simulink model "PolePlacement_Observer_DUE_SISO"  (R2019a)
settings: Solver=FixedStepAuto  StartTime=0.0  StopTime=120  RelTol=1e-3  EnableMultiTasking=on
undefined symbols (not defined in the file): A, B, C, DiscIntNeverNeededParam, i0, K, L, sigbuilder_block, Ts, u0, y0
libraries: arduinolib x1
settings Model: SimulationMode=external  ExtModeTrigDuration=2  Creator=jakub  LastModifiedBy=jakub
settings OptimizationCC: EnhancedBackFolding=on  PassReuseOutputArgsAs=Individual arguments  MaxStackSize=64  OptimizeBlockOrder=speed  DifferentSizesBufferReuse=on  OptimizationCustomize=off
settings DebuggingCC: ParameterTunabilityLossMsg=error
settings HardwareCC: ProdBitPerPointer=32  ProdBitPerSizeT=32  ProdBitPerPtrDiffT=32  ProdLargestAtomicInteger=Long  ProdLargestAtomicFloat=Double  ProdWordSize=32  ProdHWDeviceType=ARM Compatible->ARM Cortex
settings SFSimCC: MATLABDynamicMemAlloc=off
settings RTWCC: SystemTargetFile=ert.tlc  HardwareBoard=Arduino Due  TLCOptions=-aInlineSetEventsForThisBaseRateFcn=TLC_FALSE -aSuppressMultiTaskScheduler=TLC_FALSE -aRateBasedStepFcn=1  TemplateMakefile=ert_default_tmf  GenerateReport=on  Toolchain=Arduino ARM  BuildConfiguration=Faster Runs  IncludeHyperlinkInReport=on  LaunchReport=on  GenerateTraceInfo=on  GenerateTraceReport=on  GenerateTraceReportSl=on  GenerateTraceReportSf=on  GenerateTraceReportEml=on
settings CodeAppCC: ForceParamTrailComments=on  IgnoreCustomStorageClasses=off  OperatorAnnotations=on  SimulinkDataObjDesc=on  SFDataObjDesc=on  InsertBlockDesc=on
settings ERTTargetCC: SupportContinuousTime=on  SupportVariableSizeSignals=on  ExtModeStaticAllocSize=24576

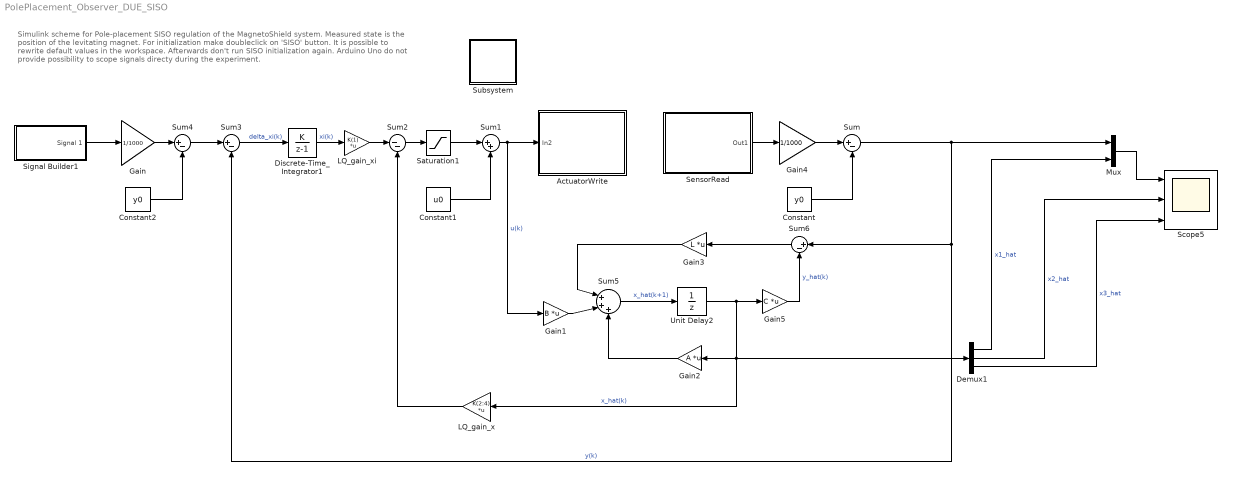
== system PolePlacement_Observer_DUE_SISO ==
  note: Simulink scheme for Pole-placement SISO regulation of the MagnetoShield system. Measured state is the position
      | of the levitating magnet.
      | For initialization make doubleclick on 'SISO' button.
      |
      | It is possible to rewrite default values in the workspace. Afterwards don't run SISO initialization again.
      |
      | Arduino Uno do not provide possibility to scope signals directy during the experiment.
  ActuatorWrite : Subsystem  AncestorBlock=MagnetoLibrary/ActuatorWrite  mask{Board=DUE, Units=Volts}
      mask prompts: Board "Type of the Arduino board"; Units "Input unite"
      mask help:
      | ActuatorWrite block allows to set desired voltage value on the electromagnet.
      | Input signal:
      |  - Voltage - value in range 0 - 12 V
      |  - Percent
      |  - DAC levels - value in range 0 - 4095
      | This block converts input control signal into suficient form (12-bit number) and writes the information on the MCP4725-DAC converter.
      mask init:
      | mask_popup = get_param(gcb,'Board'); % which popup is choosen
      | % path to the I2C Write block
      | system = gcb;
      | way = strcat(system,'/I2C Write UNO');
      | % set Module based on Arduino type
      | if strcmp(mask_popup(1),'U')
      |     set_param(way,'I2CModule','0'); % Uno/Mega - module 0
      | elseif strcmp(mask_popup(1),'D')
      |     set_param(way,'I2CModule','1'); % Due - module 1
      | end
      settings: CopyFcn=set_param(gcb, 'LinkStatus', 'inactive')
      mask TypeOptions Board: UNO/MEGA | DUE
      mask TypeOptions Units: Volts | Percent | DAC levels
      mask DialogControl DescGroupVar Prompt: ActuatorWrite block
      mask DialogControl Container3 Prompt: Arduino board
      mask Display: image('assets\MagnetoFig\ActuatorWrite.svg');
  Constant : Constant  Value=y0
  Constant1 : Constant  Value=u0
  Constant2 : Constant  Value=y0
  Demux1 : Demux  Outputs=3
  Discrete-Time_ Integrator1 : DiscreteIntegrator  IntegratorMethod=Accumulation: Forward Euler  SampleTime=Ts  LimitOutput=on  UpperSaturationLimit=1  LowerSaturationLimit=-1  ICPrevOutput=DiscIntNeverNeededParam  ICPrevScaledInput=DiscIntNeverNeededParam
  Gain : Gain  Gain=1/1000
  Gain1 : Gain  Gain=B  Multiplication=Matrix(K*u)
  Gain2 : Gain  Gain=A  Multiplication=Matrix(K*u)
  Gain3 : Gain  Gain=L  Multiplication=Matrix(K*u)
  Gain4 : Gain  Gain=1/1000
  Gain5 : Gain  Gain=C  Multiplication=Matrix(K*u)
  LQ_gain_x : Gain  Gain=K(2:4)  Multiplication=Matrix(K*u)
  LQ_gain_xi : Gain  Gain=K(1)  Multiplication=Matrix(K*u)
  Mux : Mux  Inputs=2
  Saturation1 : Saturate  UpperLimit=12-u0  LowerLimit=0-u0
  Scope5 : Scope  NumInputPorts=3
  SensorRead : Subsystem  AncestorBlock=MagnetoLibrary/SensorRead  mask{board=DUE, sensor=Distance [mm], sampling=Ts}
      mask prompts: board "Type of the Arduino board"; sensor "Sensor type"; sampling "Sampling period [s]"
      mask help: Output of the block provides data about a choosen quantity measured on the MagnetoShiled device.
      mask init:
      | letter = sensor;
      | if letter==1 % distance
      | path='assets\MagnetoFig\SensorRead\SensorRead_Hall.svg';
      | elseif letter==2 % current
      | path='assets\MagnetoFig\SensorRead\SensorRead_Current.svg';
      | elseif letter==3 % voltage
      | path='assets\MagnetoFig\SensorRead\SensorRead_Voltage.svg';
      | else % reference
      | path='assets\MagnetoFig\SensorRead\Potentiometer.svg';    
      | end
      settings: CopyFcn=set_param(gcb, 'LinkStatus', 'inactive')
      mask TypeOptions board: UNO/MEGA | DUE
      mask TypeOptions sensor: Distance [mm] | Current [mA] | Voltage [V] | Analog reference [%]
      mask Callback sensor:
      | mask_popup = get_param(gcb,'sensor'); % which popup is choosen
      | % path to the I2C Write block
      | system = gcb;
      | way = strcat(system,'/Analog Input');
      | % set Module based on Arduino type
      | if strcmp(mask_popup(1),'D')
      |     set_param(way,'pinNumber','3');
      | elseif strcmp(mask_popup(1),'V')
      |     set_param(way,'pinNumber','1'); % Due - module 1
      | elseif strcmp(mask_popup(1),'C')
      |     set_param(way,'pinNumber','2'); % Due - module 1
      | elseif strcmp(mask_popup(1),'A')
      |     set_param(way,'pinNumber','0'); % Due - module 11
      | end
      mask DialogControl DescGroupVar Prompt: SensorRead block
      mask DialogControl Container3 Prompt: Arduino board
      mask Display: image(path);
  Signal Builder1 : Subsystem  Tag=STV Subsys  LoadFcn=sigbuilder_block('load');  StartFcn=sigbuilder_block('start');  StopFcn=sigbuilder_block('stop');  ClipboardFcn=sigbuilder_block('clipboard');  mask(Sigbuilder block){tuvar=[0:10]}
      mask help: Simulink:masks:SigbuilderBlock_MD
      mask init:
      | if ~strcmp(get_param(bdroot(gcbh),'SimulationStatus'),'stopped') tuvar = sigbuilder_block('maskInit'); end
      settings: CopyFcn=sigbuilder_block('copy');  DeleteFcn=sigbuilder_block('delete');  ModelCloseFcn=sigbuilder_block('modelClose');  PreSaveFcn=sigbuilder_block('preSave');  PauseFcn=sigbuilder_block('pause');  ContinueFcn=sigbuilder_block('continue');  NameChangeFcn=sigbuilder_block('namechange');  OpenFcn=sigbuilder_block('open',[61.8 52.2 1012.8 447.6 ]);  CloseFcn=sigbuilder_block('close');
      mask Display: plot(0, 0, 100, 100,[2, 2, 32, 32, 2], [68, 8, 8, 68, 68],[32, 2], [38, 38], [32, 19, 2],[53, 60, 44], [32, 17, 17, 2],[16, 16, 31, 31]);txt = getActiveGroup(gcbh);text(2, 100, txt,'verticalAlignment', 'top');
  Subsystem : Subsystem
      settings: OpenFcn=|
      | clear;close all;clc;
      | load '../../../../matlab/examples/MagnetoShield/MagnetoShield_Models_Greybox_SS';
      | %% MagnetoShield - Pole-placement simulation and control initialization for Simulink
      | Ts = 0.001;                   % Sampling of the Simulink simulation
      | 
      | % Matrices extraction from model
      | modeld=c2d(model,Ts);           % Discretized linear state-space model
      | A = modeld.a;                   % Extract A
      | B = modeld.b;                   % Extract B
      | C = [1 0 0];                   % Position is measured for integrator 'xi' computation
      | 
      | % Discrete augmented model with integrator state - unstable, unobservable
      | Ai = [1 -C;
      |       zeros(3,1) A];
      | Bi = [0;B];
      | 
      | % Observer gain L computation
      | polesL = [-0.003 0.0006715 -0.00003715]; % desired poles of observer
      | p = poly(polesL);                        % polynomial coeficients
      | I = eye(size(A));
      | phy = p(4)*I+p(3)*A+p(2)*A^2+A^3;
      | L = phy*inv([C; C*A; C*A^2])*[0 0 1]';   % Ackermann's formula for observer
      | 
      | % Pole-placement gain K for augmented system
      | polesK = [0.985 0.5353 0.826 0.9581];       % desired poles of the system
      | p = poly(polesK);                           % polynomial coeficients
      | I = eye(size(Ai));
      | phy = p(5)*I+p(4)*Ai+p(3)*Ai^2+p(2)*Ai^3+Ai^4;
      | K = [0 0 0 1]*inv([Bi Ai*Bi Ai^2*Bi Ai^3*Bi])*phy; % Ackermann's formula for gain K
      mask Display: disp('SISO')
  Sum{,3..4,6} (4 alike) : Sum  Inputs=|+-
  Sum1 : Sum  Inputs=|++
  Sum2 : Sum  Inputs=|--
  Sum5 : Sum  Inputs=|+++
  Unit Delay2 : UnitDelay  InitialCondition=[0.017-y0;0;0-i0]  SampleTime=-1  HasFrameUpgradeWarning=on
  wires:
  Constant2/1 -> Sum4/2
  LQ_gain_xi/1 -> Sum2/1
  Discrete-Time_ Integrator1/1 -> LQ_gain_xi/1  "xi(k)"
  Gain/1 -> Sum4/1
  Gain1/1 -> Sum5/2
  Unit Delay2/1 -> Gain5/1, Demux1/1, Gain2/1, LQ_gain_x/1  "x_hat(k)"
  LQ_gain_x/1 -> Sum2/2
  Saturation1/1 -> Sum1/1
  Sum4/1 -> Sum3/1
  Sum6/1 -> Gain3/1
  Gain5/1 -> Sum6/2  "y_hat(k)"
  Constant1/1 -> Sum1/2
  Sum1/1 -> Gain1/1, ActuatorWrite/1(In2)  "u(k)"
  Constant/1 -> Sum/2
  Gain2/1 -> Sum5/3
  Sum5/1 -> Unit Delay2/1  "x_hat(k+1)"
  SensorRead/1(Out1) -> Gain4/1
  Gain3/1 -> Sum5/1
  Sum2/1 -> Saturation1/1
  Sum3/1 -> Discrete-Time_ Integrator1/1  "delta_xi(k)"
  Gain4/1 -> Sum/1
  Signal Builder1/1(Signal 1) -> Gain/1
  Demux1/2 -> Scope5/2  "x2_hat"
  Demux1/1 -> Mux/2  "x1_hat"
  Mux/1 -> Scope5/1
  Sum/1 -> Sum3/2, Sum6/1, Mux/1  "y(k)"
  Demux1/3 -> Scope5/3  "x3_hat"

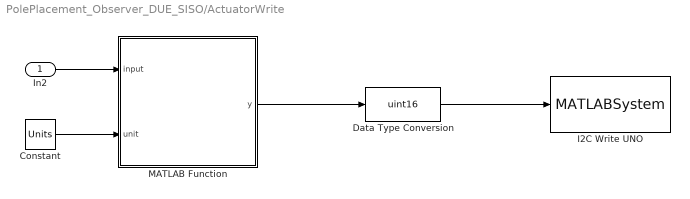
== system PolePlacement_Observer_DUE_SISO/ActuatorWrite ==
  In2 : Inport
  Constant : Constant  Value=Units
  Data Type Conversion : DataTypeConversion  OutDataTypeStr=uint16
  I2C Write UNO : MATLABSystem  AncestorBlock=arduinolib/I2C Write  InitFcn=|  System=codertarget.arduinobase.internal.arduinoI2CWrite  I2CModule=1  Mode=Master  SlaveAddress=96  SlaveByteOrder=BigEndian  Direction=Transmitter  RegisterAddressMode=off  RegisterAddress=0  SlaveDataType=uint8  DataLength=1  NoAck=off  RepeatedStart=off  OutputStatus=off  blockPlatform=ARDUINO
      | codertarget.arduinobase.blocks.registerI2CBlock(gcbh);
      | codertarget.arduinobase.blocks.arduinoBlockInitFcnCallback(gcbh);
      mask Type: I2C Write
      mask Display:
      | color('white');
      | plot([100,100,100,100],[100,100,100,100]);
      | plot([0,0,0,0],[0,0,0,0]);
      | color('blue');
      | text(99, 92, 'ARDUINO', 'horizontalAlignment', 'right');
      | color('black');
      | text(50,60,'\fontsize{12}\bfI2C','texmode','on','horizontalAlignment','center','verticalAlignment','middle');
      | text(50,40,'\fontsize{10}\bfMaster Write','texmode','on','horizontalAlignment','center','verticalAlignment','middle');
      | text(50,15,'Slave: 0x60' ,'horizontalAlignment', 'center');
      | port_label('input',1,'Data');
  MATLAB Function : MATLAB Function  TreatAsAtomicUnit=on
  wires:
  MATLAB Function/1(y) -> Data Type Conversion/1
  Data Type Conversion/1 -> I2C Write UNO/1
  Constant/1 -> MATLAB Function/2(unit)
  In2/1 -> MATLAB Function/1(input)

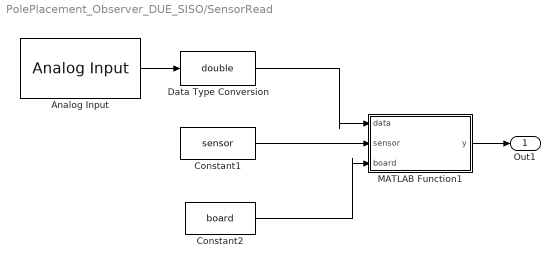
== system PolePlacement_Observer_DUE_SISO/SensorRead ==
  Analog Input : arduinolib/Analog Input  pinNumber=3  ReadResultsOnly=off  ConversionTriggerSource=Software  ExternalTriggerType=uint32(0)  OutputDataType=uint16  EnableConversionCompleteNotify=off  EnableOuputStatus=off  SampleTime=sampling  blockPlatform=arduino
  Constant1 : Constant  Value=sensor
  Constant2 : Constant  Value=board
  Data Type Conversion : DataTypeConversion  OutDataTypeStr=double
  MATLAB Function1 : MATLAB Function  TreatAsAtomicUnit=on
  Out1 : Outport
  wires:
  Analog Input/1 -> Data Type Conversion/1
  Data Type Conversion/1 -> MATLAB Function1/1(data)
  MATLAB Function1/1(y) -> Out1/1
  Constant1/1 -> MATLAB Function1/2(sensor)
  Constant2/1 -> MATLAB Function1/3(board)

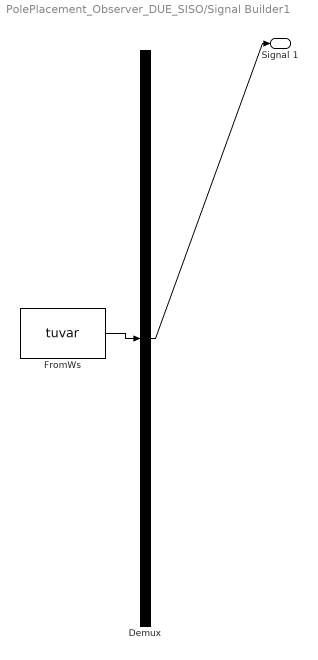
== system PolePlacement_Observer_DUE_SISO/Signal Builder1 ==
  Demux : Demux  Tag=STV Demux  Outputs=1
  FromWs : FromWorkspace  Tag=STV FromWs  VariableName=tuvar  SampleTime=0
      SigBuilderData=|
      | common.afterFinalStr = 'Extrapolate'
      | common.sampleTime = 0
      | dataSet.timeRange = [0 120]
      | dataSet.name = 'Group 1'
      | sbobj.Groups.Name = 'Group 1'
      | sbobj.Groups.Signals.Name = 'Signal 1'
      | sbobj.Groups.Signals.XData = [0 5 5 10 15 15 20 25 25 30 35 35 40 45 45 50 55 55 60 65 70 70 75 80 85 85 90 95 100 105 110 115 115 120]
      | sbobj.Groups.Signals.YData = [17 17 16.5 16.5 16.5 15.5 15.5 15.5 14.5 14.5 14.5 13.5 13.5 13.5 12.5 12.5 12.5 16 16 16 16 13.5 13.5 13.5 13.5 15 15 15 17 12 14.5 14.5 17 17]
      | sbobj.Groups.TimeRange = [0 120]
  Signal 1 : Outport  Tag=STV Outport
  wires:
  FromWs/1 -> Demux/1
  Demux/1 -> Signal 1/1

== system PolePlacement_Observer_DUE_SISO/Subsystem ==

== matlab function PolePlacement_Observer_DUE_SISO/ActuatorWrite/MATLAB Function ==
  data: input input; y output; unit input
function y = fcn(input,unit)

if unit==1 % voltage
    y = 4095/12*input;
elseif unit==2 % percents
    y = 4095/100*input;
elseif unit==3 % dac levels
    y = input;
else
     y = 0; % needed instance
end
% secures that 12-bit number will not overcross a size boundary
if y>4095
    y=4095;
elseif y<0
    y=0;
end

end

== matlab function PolePlacement_Observer_DUE_SISO/SensorRead/MATLAB Function1 ==
  data: data input; y output; sensor input; board input
function y = fcn(data,sensor,board)
persistent init A1302_SENSITIVITY Dconst1 Dconst2 I_gain V_gain ARES3V3;
if isempty(init)
    init = 1;
    A1302_SENSITIVITY = 769.23;
    Dconst1 = 3.233100;
    Dconst2 = 0.220571;
    I_gain = 33.333333;
    V_gain = 4;
    if board==1
        ARES3V3 = 3.3/1023; % ADC constant for AVR architecture
    else
        ARES3V3 = 3.3/4095; % ADC constant for SAM/SAMD architecture
    end
end

if sensor==1                    % position
    gauss = (2.5-data*ARES3V3)*A1302_SENSITIVITY;
    y = Dconst1*gauss^Dconst2;
elseif sensor==2                % current
    y = data*ARES3V3*I_gain;
elseif sensor==3                % voltage
    y = data*ARES3V3*V_gain;
else                            % analog reference
    y = data*ARES3V3*100/3.3;
end
